simulink model "test02_sensor"  (R2013b)
settings: Solver=FixedStepDiscrete  StartTime=0.0  StopTime=10.0  FixedStep=0.05  RelTol=1e-3
InitFcn:
  | load 'variabili.mat'
values from neighbouring files (symbols this model uses):
  var = [0,45,90]    [variabili.m]    (also in variabili.mat = [0 45 90])
  var2 = [0.5,3.6,4.5]    [variabili.m]    (also in variabili.mat = [0.5 3.6 4.5])
undefined symbols (not defined in the file or in its folder): sigbuilder_block
settings Model: Creator=training-it  LastModifiedBy=training-it

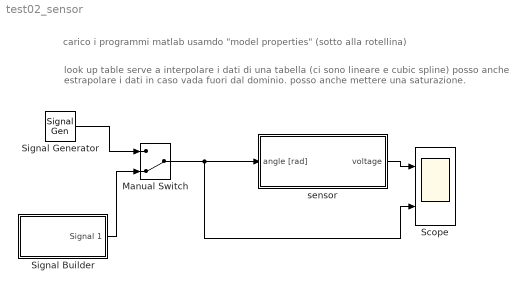
== system test02_sensor ==
  note: look up table serve a interpolare i dati di una tabella (ci sono lineare e cubic spline)
      | posso anche estrapolare i dati in caso vada fuori dal dominio. posso anche mettere una saturazione.
  note: carico i programmi matlab usamdo "model properties" (sotto alla rotellina)
  Manual Switch : ManualSwitch  CurrentSetting=0
  Scope : Scope  NumInputPorts=2
      settings: YMin=-5~-5  YMax=5~5
  Signal Generator : SignalGenerator  WaveForm=sawtooth  Amplitude=pi/2
  Signal Builder : Subsystem  Tag=STV Subsys  LoadFcn=sigbuilder_block('load');  StartFcn=sigbuilder_block('start');  StopFcn=sigbuilder_block('stop');  ClipboardFcn=sigbuilder_block('clipboard');  mask(Sigbuilder block){}
      mask help: Simulink:masks:SigbuilderBlock_MD
      mask init:
      | if ~strcmp(get_param(bdroot(gcbh),'SimulationStatus'),'stopped') tuvar = sigbuilder_block('maskInit'); end
      settings: CopyFcn=sigbuilder_block('copy');  DeleteFcn=sigbuilder_block('delete');  ModelCloseFcn=sigbuilder_block('modelClose');  PreSaveFcn=sigbuilder_block('preSave');  PauseFcn=sigbuilder_block('pause');  ContinueFcn=sigbuilder_block('continue');  NameChangeFcn=sigbuilder_block('namechange');  OpenFcn=sigbuilder_block('open',[437.25 199.5 550.5 399.75 ]);  CloseFcn=sigbuilder_block('close');
      mask Display: plot(0, 0, 100, 100,[2, 2, 32, 32, 2], [68, 8, 8, 68, 68],[32, 2], [38, 38], [32, 19, 2],[53, 60, 44], [32, 17, 17, 2],[16, 16, 31, 31]);txt = getActiveGroup(gcbh);text(2, 100, txt,'verticalAlignment', 'top');
  sensor : Subsystem
  wires:
  sensor/1(voltage) -> Scope/1
  Manual Switch/1 -> Scope/2, sensor/1(angle [rad])
  Signal Builder/1(Signal 1) -> Manual Switch/2
  Signal Generator/1 -> Manual Switch/1

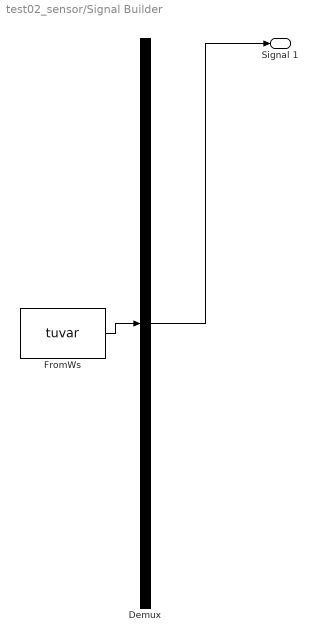
== system test02_sensor/Signal Builder ==
  Demux : Demux  Tag=STV Demux  Outputs=1
  FromWs : FromWorkspace  Tag=STV FromWs  VariableName=tuvar  SampleTime=0
      SigBuilderData=|
      | common.afterFinalStr = 'Extrapolate'
      | common.sampleTime = 0
      | dataSet(1).timeRange = [0 10]
      | dataSet(1).name = 'Accelerazione'
      | dataSet(2).timeRange = [0 10]
      | dataSet(2).name = 'Accelerazione2_HardStop'
      | sbobj.Groups(1).Name = 'Accelerazione'
      | sbobj.Groups(1).Signals.Name = 'Signal 1'
      | sbobj.Groups(1).Signals.XData = [0 1.98 2.98 4 4.7 6 6.94 10]
      | sbobj.Groups(1).Signals.YData = [0.02 0.006 0.4 0.41 1.57079632679 1.58 0.004 0]
      | sbobj.Groups(2).Name = 'Accelerazione2_HardStop'
      | sbobj.Groups(2).Signals.Name = 'Signal 1'
      | sbobj.Groups(2).Signals.XData = [0 1.98 2.98 4 4.7 6 6.94 10]
      | sbobj.Groups(2).Signals.YData = [1.49 1.49 -0.01 0 0.01 0.02 0.004 0]
  Signal 1 : Outport  Tag=STV Outport
  wires:
  Demux/1 -> Signal 1/1
  FromWs/1 -> Demux/1

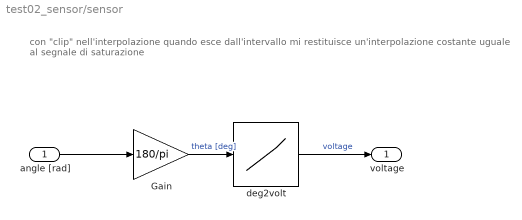
== system test02_sensor/sensor ==
  note: con "clip" nell'interpolazione quando esce dall'intervallo mi restituisce un'interpolazione costante uguale al segnale di saturazione
  angle [rad] : Inport
  Gain : Gain  Gain=180/pi
  deg2volt : Lookup_n-D  NumberOfTableDimensions=1  BreakpointsForDimension1=var  Table=var2  TableMin=[0.5]  TableMax=[4.5]  ExtrapMethod=Clip  InternalRulePriority=Speed  RndMeth=Simplest  InputSameDT=on
  voltage : Outport
  wires:
  angle [rad]/1 -> Gain/1
  Gain/1 -> deg2volt/1  "theta [deg]"
  deg2volt/1 -> voltage/1  "voltage"
